simulink model "Assign1_3K04"  (R2022a)
settings: Solver=FixedStepAuto  StartTime=0.0  StopTime=10.0  FixedStep=1e-3  RelTol=1e-3  EnableMultiTasking=on
settings Model: ExtModeTrigDuration=5  Creator=sabri  LastModifiedBy=Tim
settings SolverCC: AlgebraicLoopSolver=TrustRegion
settings OptimizationCC: EnhancedBackFolding=on  PassReuseOutputArgsAs=Individual arguments  ZeroExternalMemoryAtStartup=off  ZeroInternalMemoryAtStartup=off  MaxStackSize=64  OptimizeBlockOrder=speed  DifferentSizesBufferReuse=on  OptimizationCustomize=off  EfficientTunableParamExpr=on
settings DebuggingCC: ParameterTunabilityLossMsg=error  UnconnectedInputMsg=warning  UnconnectedOutputMsg=warning  UnconnectedLineMsg=warning  SFMachineParentedDataDiag=warning
settings HardwareCC: ProdBitPerPointer=32  ProdBitPerSizeT=32  ProdBitPerPtrDiffT=32  ProdLargestAtomicInteger=Long  ProdLargestAtomicFloat=Double  ProdWordSize=32  ProdHWDeviceType=ARM Compatible->ARM Cortex
settings SFSimCC: MATLABDynamicMemAlloc=off
settings RTWCC: SystemTargetFile=ert.tlc  HardwareBoard=NXP FRDM-K64F  TLCOptions="-aInlineSetEventsForThisBaseRateFcn=TLC_FALSE -aSuppressMultiTaskScheduler=TLC_FALSE  -aRateBasedStepFcn=0"  TemplateMakefile=ert_default_tmf  Toolchain=GNU Tools for ARM Embedded Processors
settings CodeAppCC: ForceParamTrailComments=on  IgnoreCustomStorageClasses=off  OperatorAnnotations=on  SimulinkDataObjDesc=on  SFDataObjDesc=on  InsertBlockDesc=on

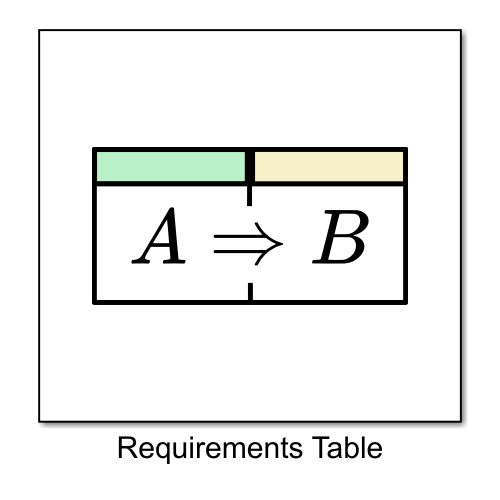
[thumbnail: Simulink's stored preview of the top-level diagram]
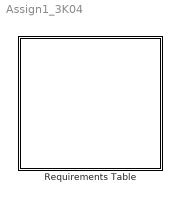
== system Assign1_3K04 ==
  Requirements Table : Requirements Table  TreatAsAtomicUnit=on

== stateflow chart Assign1_3K04/Requirements Table ==
  (default) -> (junction 1073743612)
  (junction 1073743612) -> (junction 1073743613) : {
      | % SF_REQ_REV_07
      | }
  (junction 1073743613) -> (junction 1073743615) : {
      | % HEADER_ASSIGNMENTS
      |
      | }
  (junction 1073743615) -> (junction 1073743617) : {
      | % START_A_4
      | }
  (junction 1073743617) -> (junction 1073743619) : {
      | }
  (junction 1073743619) -> (junction 1073743621)
  (junction 1073743621) -> (junction 1073743623) : {
      | }
  (junction 1073743623) -> (junction 1073743625) : {
      | % END_A_4
      | }
  (junction 1073743625) -> (junction 1073743627) : {
      | % START_R_1
      | }
  (junction 1073743627) -> (junction 1073743629) : {
      | }
  (junction 1073743629) -> (junction 1073743631)
  (junction 1073743631) -> (junction 1073743633) [order 1] : [(((MODE) == (1)))]
  (junction 1073743631) -> (junction 1073743675) [order 2]
  (junction 1073743633) -> (junction 1073743635) : {
      | reqtable_postcondition((((FRONTEND_CTRL) == (0))), 'R:1');
      |
      |
      | }
  (junction 1073743635) -> (junction 1073743637) : {
      | }
  (junction 1073743637) -> (junction 1073743639) : {
      | % START_R_10
      | }
  (junction 1073743639) -> (junction 1073743641) : {
      | }
  (junction 1073743641) -> (junction 1073743643)
  (junction 1073743643) -> (junction 1073743645) [order 1] : [(((STATE) == (1)))]
  (junction 1073743643) -> (junction 1073743651) [order 2]
  (junction 1073743645) -> (junction 1073743647) : {
      | reqtable_postcondition((((STATE) == (0))) && (((PACE_CHARGE_CTRL) == (0))) && (((PACE_GND_CTRL) == (1))) && (((Z_ATR_CTRL) == (0))) && (((Z _VENT_CTRL) == (0))) && (((VENT_PACE_CTRL) == (1))) && (((ATR_PACE_CTRL) == (0))) && (((VENT_GND_CTRL) == (0))) && (((ATR_GND_CTRL) == (0))), 'R:1.1');
      |
      |
      | }
  (junction 1073743647) -> (junction 1073743649) : {
      | }
  (junction 1073743649) -> (junction 1073743651)
  (junction 1073743651) -> (junction 1073743653)
  (junction 1073743653) -> (junction 1073743655) : {
      | % END_R_10
      | }
  (junction 1073743655) -> (junction 1073743657) : {
      | % START_R_16
      | }
  (junction 1073743657) -> (junction 1073743659) : {
      | }
  (junction 1073743659) -> (junction 1073743661)
  (junction 1073743661) -> (junction 1073743663) [order 1] : [(((STATE) == (0)))]
  (junction 1073743661) -> (junction 1073743669) [order 2]
  (junction 1073743663) -> (junction 1073743665) : {
      | reqtable_postcondition((((STATE) == (1))) && (((PACE_CHARGE_CTRL) == (1))) && (((PACE_GND_CTRL) == (1))) && (((Z_ATR_CTRL) == (0))) && (((Z _VENT_CTRL) == (0))) && (((VENT_PACE_CTRL) == (0))) && (((ATR_PACE_CTRL) == (0))) && (((VENT_GND_CTRL) == (1))) && (((ATR_GND_CTRL) == (0))), 'R:1.2');
      |
      |
      | }
  (junction 1073743665) -> (junction 1073743667) : {
      | }
  (junction 1073743667) -> (junction 1073743669)
  (junction 1073743669) -> (junction 1073743671)
  (junction 1073743671) -> (junction 1073743673) : {
      | % END_R_16
      | }
  (junction 1073743673) -> (junction 1073743675)
  (junction 1073743675) -> (junction 1073743677)
  (junction 1073743677) -> (junction 1073743679) : {
      | % END_R_1
      | }
  (junction 1073743679) -> (junction 1073743681) : {
      | % START_R_7
      | }
  (junction 1073743681) -> (junction 1073743683) : {
      | }
  (junction 1073743683) -> (junction 1073743685)
  (junction 1073743685) -> (junction 1073743687) [order 1] : [(((MODE) == (2)))]
  (junction 1073743685) -> (junction 1073743729) [order 2]
  (junction 1073743687) -> (junction 1073743689) : {
      | reqtable_postcondition((((FRONTEND_CTRL) == (0))), 'R:2');
      |
      |
      | }
  (junction 1073743689) -> (junction 1073743691) : {
      | }
  (junction 1073743691) -> (junction 1073743693) : {
      | % START_R_19
      | }
  (junction 1073743693) -> (junction 1073743695) : {
      | }
  (junction 1073743695) -> (junction 1073743697)
  (junction 1073743697) -> (junction 1073743699) [order 1] : [(((STATE) == (1)))]
  (junction 1073743697) -> (junction 1073743705) [order 2]
  (junction 1073743699) -> (junction 1073743701) : {
      | reqtable_postcondition((((STATE) == (0))) && (((PACE_CHARGE_CTRL) == (0))) && (((PACE_GND_CTRL) == (1))) && (((Z_ATR_CTRL) == (0))) && (((Z _VENT_CTRL) == (0))) && (((VENT_PACE_CTRL) == (0))) && (((ATR_PACE_CTRL) == (1))) && (((VENT_GND_CTRL) == (0))) && (((ATR_GND_CTRL) == (0))), 'R:2.1');
      |
      |
      | }
  (junction 1073743701) -> (junction 1073743703) : {
      | }
  (junction 1073743703) -> (junction 1073743705)
  (junction 1073743705) -> (junction 1073743707)
  (junction 1073743707) -> (junction 1073743709) : {
      | % END_R_19
      | }
  (junction 1073743709) -> (junction 1073743711) : {
      | % START_R_25
      | }
  (junction 1073743711) -> (junction 1073743713) : {
      | }
  (junction 1073743713) -> (junction 1073743715)
  (junction 1073743715) -> (junction 1073743717) [order 1] : [(((STATE) == (0)))]
  (junction 1073743715) -> (junction 1073743723) [order 2]
  (junction 1073743717) -> (junction 1073743719) : {
      | reqtable_postcondition((((STATE) == (1))) && (((PACE_CHARGE_CTRL) == (1))) && (((PACE_GND_CTRL) == (1))) && (((Z_ATR_CTRL) == (0))) && (((Z _VENT_CTRL) == (0))) && (((VENT_PACE_CTRL) == (0))) && (((ATR_PACE_CTRL) == (0))) && (((VENT_GND_CTRL) == (0))) && (((ATR_GND_CTRL) == (1))), 'R:2.2');
      |
      |
      | }
  (junction 1073743719) -> (junction 1073743721) : {
      | }
  (junction 1073743721) -> (junction 1073743723)
  (junction 1073743723) -> (junction 1073743725)
  (junction 1073743725) -> (junction 1073743727) : {
      | % END_R_25
      | }
  (junction 1073743727) -> (junction 1073743729)
  (junction 1073743729) -> (junction 1073743731)
  (junction 1073743731) -> (junction 1073743733) : {
      | % END_R_7
      | }
  (junction 1073743733) -> (junction 1073743735) : {
      | % START_R_28
      | }
  (junction 1073743735) -> (junction 1073743737) : {
      | }
  (junction 1073743737) -> (junction 1073743739)
  (junction 1073743739) -> (junction 1073743741) [order 1] : [(((MODE) == (3)))]
  (junction 1073743739) -> (junction 1073743785) [order 2]
  (junction 1073743741) -> (junction 1073743743) : {
      |
      |
      | }
  (junction 1073743743) -> (junction 1073743745) : {
      | }
  (junction 1073743745) -> (junction 1073743747) : {
      | % START_R_34
      | }
  (junction 1073743747) -> (junction 1073743749) : {
      | }
  (junction 1073743749) -> (junction 1073743751)
  (junction 1073743751) -> (junction 1073743753) [order 1] : [(((MODE) == (-threshold variable)) || ((MODE) == (sensing var)) || ((MODE) == (states change based on sensed pulse or not)))]
  (junction 1073743751) -> (junction 1073743759) [order 2]
  (junction 1073743753) -> (junction 1073743755) : {
      |
      |
      | }
  (junction 1073743755) -> (junction 1073743757) : {
      | }
  (junction 1073743757) -> (junction 1073743759)
  (junction 1073743759) -> (junction 1073743761)
  (junction 1073743761) -> (junction 1073743763) : {
      | % END_R_34
      | }
  (junction 1073743763) -> (junction 1073743765) : {
      | % START_R_37
      | }
  (junction 1073743765) -> (junction 1073743767) : {
      | }
  (junction 1073743767) -> (junction 1073743769) : {
      |
      |
      | }
  (junction 1073743769) -> (junction 1073743771) : {
      | }
  (junction 1073743771) -> (junction 1073743773) : {
      | % END_R_37
      | }
  (junction 1073743773) -> (junction 1073743775) : {
      | % START_R_40
      | }
  (junction 1073743775) -> (junction 1073743777) : {
      | }
  (junction 1073743777) -> (junction 1073743779) : {
      |
      |
      | }
  (junction 1073743779) -> (junction 1073743781) : {
      | }
  (junction 1073743781) -> (junction 1073743783) : {
      | % END_R_40
      | }
  (junction 1073743783) -> (junction 1073743785)
  (junction 1073743785) -> (junction 1073743787)
  (junction 1073743787) -> (junction 1073743789) : {
      | % END_R_28
      | }
  (junction 1073743789) -> (junction 1073743791) : {
      | % START_R_31
      | }
  (junction 1073743791) -> (junction 1073743793) : {
      | }
  (junction 1073743793) -> (junction 1073743795)
  (junction 1073743795) -> (junction 1073743797) [order 1] : [(((MODE) == (4)))]
  (junction 1073743795) -> (junction 1073743833) [order 2]
  (junction 1073743797) -> (junction 1073743799) : {
      |
      |
      | }
  (junction 1073743799) -> (junction 1073743801) : {
      | }
  (junction 1073743801) -> (junction 1073743803) : {
      | % START_R_43
      | }
  (junction 1073743803) -> (junction 1073743805) : {
      | }
  (junction 1073743805) -> (junction 1073743807) : {
      |
      |
      | }
  (junction 1073743807) -> (junction 1073743809) : {
      | }
  (junction 1073743809) -> (junction 1073743811) : {
      | % END_R_43
      | }
  (junction 1073743811) -> (junction 1073743813) : {
      | % START_R_46
      | }
  (junction 1073743813) -> (junction 1073743815) : {
      | }
  (junction 1073743815) -> (junction 1073743817) : {
      |
      |
      | }
  (junction 1073743817) -> (junction 1073743819) : {
      | }
  (junction 1073743819) -> (junction 1073743821) : {
      | % END_R_46
      | }
  (junction 1073743821) -> (junction 1073743823) : {
      | % START_R_49
      | }
  (junction 1073743823) -> (junction 1073743825) : {
      | }
  (junction 1073743825) -> (junction 1073743827) : {
      |
      |
      | }
  (junction 1073743827) -> (junction 1073743829) : {
      | }
  (junction 1073743829) -> (junction 1073743831) : {
      | % END_R_49
      | }
  (junction 1073743831) -> (junction 1073743833)
  (junction 1073743833) -> (junction 1073743835)
  (junction 1073743835) -> (junction 1073743837) : {
      | % END_R_31
      | }
